simulink model "ProposedProblem2"  (R2013a)
settings: Solver=ode45  StartTime=0.0  StopTime=1000  RelTol=1e-3
undefined symbols (not defined in the file): des, gcbh
settings Model: Creator=gabig  LastModifiedBy=gabig

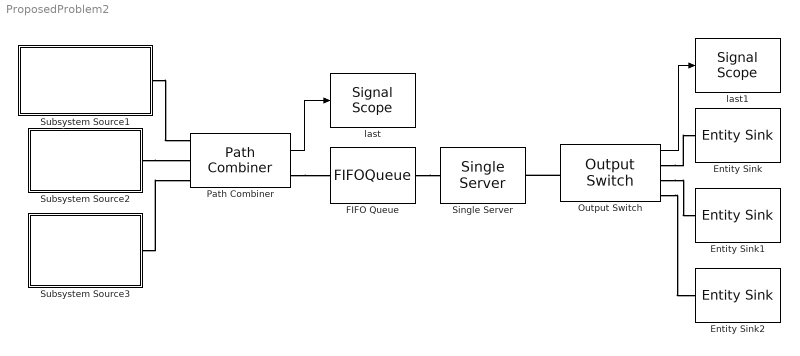
== system ProposedProblem2 ==
  Entity Sink : EntitySink
  Entity Sink1 : EntitySink
  Entity Sink2 : EntitySink
  FIFO Queue : FIFOQueue
  Output Switch : OutputSwitch  SwitchingCriterion=From attribute  AttributeName=Destination  StatLastDeparturePort=on
      settings: OutputPortMap=o3
  Path Combiner : PathCombiner  StatLastArrivalPort=on
      settings: OutputPortMap=o1
  Single Server : SingleServer
  "Subsystem Source1 " : Subsystem
  Subsystem Source2 : Subsystem
  "Subsystem Source3 " : Subsystem
  last : SignalScope  LoadFcn=des.scope.CallbackSupport('seLoadFcn',gcbh)  StartFcn=des.scope.CallbackSupport('seStartFcn',gcbh)  StopFcn=des.scope.CallbackSupport('seStopFcn',gcbh)
      settings: CopyFcn=des.scope.CallbackSupport('seCopyFcn',gcbh)  DeleteFcn=des.scope.CallbackSupport('seDeleteFcn',gcbh)  PreSaveFcn=des.scope.CallbackSupport('sePreSaveFcn',gcbh)  NameChangeFcn=des.scope.CallbackSupport('seNameChangeFcn',gcbh)  OpenFcn=des.scope.CallbackSupport('seOpenFcn',gcbh)
  last1 : SignalScope  LoadFcn=des.scope.CallbackSupport('seLoadFcn',gcbh)  StartFcn=des.scope.CallbackSupport('seStartFcn',gcbh)  StopFcn=des.scope.CallbackSupport('seStopFcn',gcbh)
      settings: CopyFcn=des.scope.CallbackSupport('seCopyFcn',gcbh)  DeleteFcn=des.scope.CallbackSupport('seDeleteFcn',gcbh)  PreSaveFcn=des.scope.CallbackSupport('sePreSaveFcn',gcbh)  NameChangeFcn=des.scope.CallbackSupport('seNameChangeFcn',gcbh)  OpenFcn=des.scope.CallbackSupport('seOpenFcn',gcbh)
  wires:
  Output Switch/1 -> last1/1
  Path Combiner/1 -> last/1
  connections:
  Output Switch/RConn2 -- Entity Sink1/LConn1
  "Subsystem Source3 "/RConn1 -- Path Combiner/LConn3
  "Subsystem Source1 "/RConn1 -- Path Combiner/LConn1
  Path Combiner/RConn1 -- FIFO Queue/LConn1
  Output Switch/LConn1 -- Single Server/RConn1
  FIFO Queue/RConn1 -- Single Server/LConn1
  Output Switch/RConn1 -- Entity Sink/LConn1
  Output Switch/RConn3 -- Entity Sink2/LConn1
  Subsystem Source2/RConn1 -- Path Combiner/LConn2

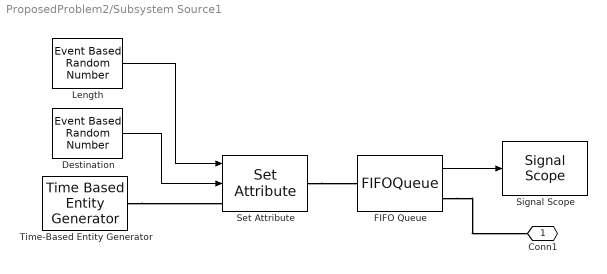
== system ProposedProblem2/Subsystem Source1  ==
  Destination : EventBasedRandomNumber  Distribution=Discrete uniform  minUnid=1  maxUnid=3  numValueUnid=3  Seed=12346
  FIFO Queue : FIFOQueue  StatNumberDeparted=on
  Length : EventBasedRandomNumber  Distribution=Discrete uniform  minUnid=6  maxUnid=10  numValueUnid=5
  Set Attribute : SetAttribute  AttributeName=Length|Destination  AttributeFrom=Signal port|Signal port  AttributeValue=1|1  AttributeTreatAsVector=1|1  EvaluatedAttributeValue={ [];[]}
      settings: InputPortMap=u0,u1
  Signal Scope : SignalScope  LoadFcn=des.scope.CallbackSupport('seLoadFcn',gcbh)  StartFcn=des.scope.CallbackSupport('seStartFcn',gcbh)  StopFcn=des.scope.CallbackSupport('seStopFcn',gcbh)
      settings: CopyFcn=des.scope.CallbackSupport('seCopyFcn',gcbh)  DeleteFcn=des.scope.CallbackSupport('seDeleteFcn',gcbh)  PreSaveFcn=des.scope.CallbackSupport('sePreSaveFcn',gcbh)  NameChangeFcn=des.scope.CallbackSupport('seNameChangeFcn',gcbh)  OpenFcn=des.scope.CallbackSupport('seOpenFcn',gcbh)
  Time-Based Entity Generator : TimeBasedEntityGenerator  Distribution=Exponential  InitialSeed=12333  Mean=8
  Conn1 : PMIOPort  Port=1  Side=Right
  wires:
  Length/1 -> Set Attribute/1
  Destination/1 -> Set Attribute/2
  FIFO Queue/1 -> Signal Scope/1
  connections:
  Set Attribute/RConn1 -- FIFO Queue/LConn1
  FIFO Queue/RConn1 -- Conn1/RConn1
  Time-Based Entity Generator/RConn1 -- Set Attribute/LConn1

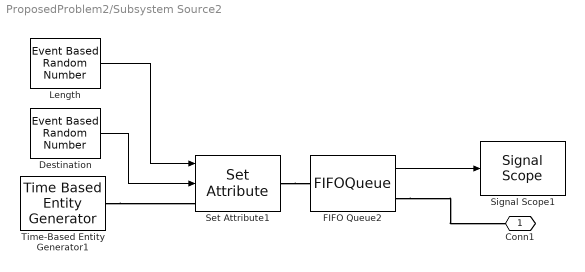
== system ProposedProblem2/Subsystem Source2 ==
  " Destination " : EventBasedRandomNumber  Distribution=Discrete uniform  minUnid=1  maxUnid=3  numValueUnid=3  Seed=12348
  " Length" : EventBasedRandomNumber  Distribution=Discrete uniform  minUnid=6  maxUnid=10  numValueUnid=5  Seed=12347
  FIFO Queue2 : FIFOQueue  StatNumberDeparted=on
  Set Attribute1 : SetAttribute  AttributeName=Length|Destination  AttributeFrom=Signal port|Signal port  AttributeValue=1|1  AttributeTreatAsVector=1|1  EvaluatedAttributeValue={ [];[]}
      settings: InputPortMap=u0,u1
  Signal Scope1 : SignalScope  LoadFcn=des.scope.CallbackSupport('seLoadFcn',gcbh)  StartFcn=des.scope.CallbackSupport('seStartFcn',gcbh)  StopFcn=des.scope.CallbackSupport('seStopFcn',gcbh)
      settings: CopyFcn=des.scope.CallbackSupport('seCopyFcn',gcbh)  DeleteFcn=des.scope.CallbackSupport('seDeleteFcn',gcbh)  PreSaveFcn=des.scope.CallbackSupport('sePreSaveFcn',gcbh)  NameChangeFcn=des.scope.CallbackSupport('seNameChangeFcn',gcbh)  OpenFcn=des.scope.CallbackSupport('seOpenFcn',gcbh)
  Time-Based Entity Generator1 : TimeBasedEntityGenerator  Distribution=Exponential  InitialSeed=12333  Mean=8
  Conn1 : PMIOPort  Port=1  Side=Right
  wires:
  " Length"/1 -> Set Attribute1/1
  " Destination "/1 -> Set Attribute1/2
  FIFO Queue2/1 -> Signal Scope1/1
  connections:
  Set Attribute1/RConn1 -- FIFO Queue2/LConn1
  FIFO Queue2/RConn1 -- Conn1/RConn1
  Time-Based Entity Generator1/RConn1 -- Set Attribute1/LConn1

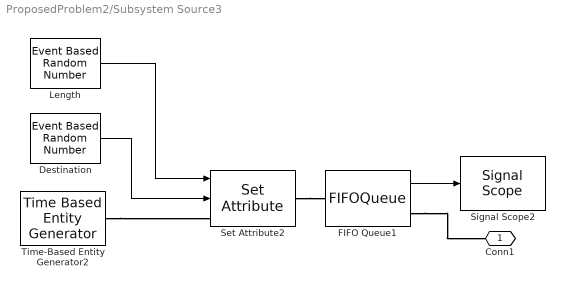
== system ProposedProblem2/Subsystem Source3  ==
  Destination : EventBasedRandomNumber  Distribution=Discrete uniform  minUnid=1  maxUnid=3  numValueUnid=3  Seed=12310
  FIFO Queue1 : FIFOQueue  StatNumberDeparted=on
  Length : EventBasedRandomNumber  Distribution=Discrete uniform  minUnid=6  maxUnid=10  numValueUnid=5  Seed=12349
  Set Attribute2 : SetAttribute  AttributeName=Length|Destination  AttributeFrom=Signal port|Signal port  AttributeValue=1|1  AttributeTreatAsVector=1|1  EvaluatedAttributeValue={ [];[]}
      settings: InputPortMap=u0,u1
  Signal Scope2 : SignalScope  LoadFcn=des.scope.CallbackSupport('seLoadFcn',gcbh)  StartFcn=des.scope.CallbackSupport('seStartFcn',gcbh)  StopFcn=des.scope.CallbackSupport('seStopFcn',gcbh)
      settings: CopyFcn=des.scope.CallbackSupport('seCopyFcn',gcbh)  DeleteFcn=des.scope.CallbackSupport('seDeleteFcn',gcbh)  PreSaveFcn=des.scope.CallbackSupport('sePreSaveFcn',gcbh)  NameChangeFcn=des.scope.CallbackSupport('seNameChangeFcn',gcbh)  OpenFcn=des.scope.CallbackSupport('seOpenFcn',gcbh)
  Time-Based Entity Generator2 : TimeBasedEntityGenerator  Distribution=Exponential  InitialSeed=12333  Mean=8
  Conn1 : PMIOPort  Port=1  Side=Right
  wires:
  Length/1 -> Set Attribute2/1
  Destination/1 -> Set Attribute2/2
  FIFO Queue1/1 -> Signal Scope2/1
  connections:
  Time-Based Entity Generator2/RConn1 -- Set Attribute2/LConn1
  Set Attribute2/RConn1 -- FIFO Queue1/LConn1
  FIFO Queue1/RConn1 -- Conn1/RConn1
